simulink model "SimpleOrbitModel"  (R2025b)
settings: Solver=ode4  StartTime=0.0  StopTime=20000  FixedStep=60  RelTol=1e-3
undefined symbols (not defined in the file or in its folder): IAU, juliandate
libraries: aerolibtransform2 x1, aerolibatmos2 x1
settings Model: Creator=mbgm9nc4  LastModifiedBy=ewanb

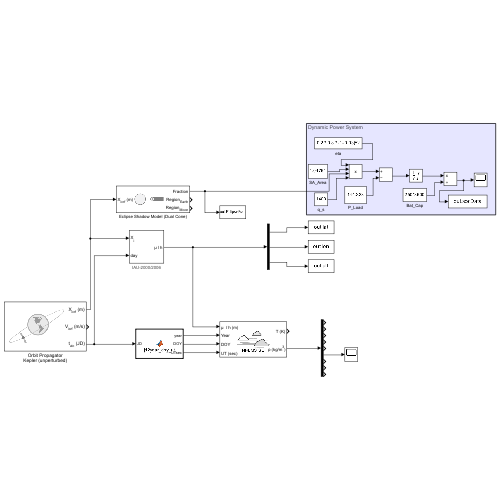
[thumbnail: Simulink's stored preview of the top-level diagram]
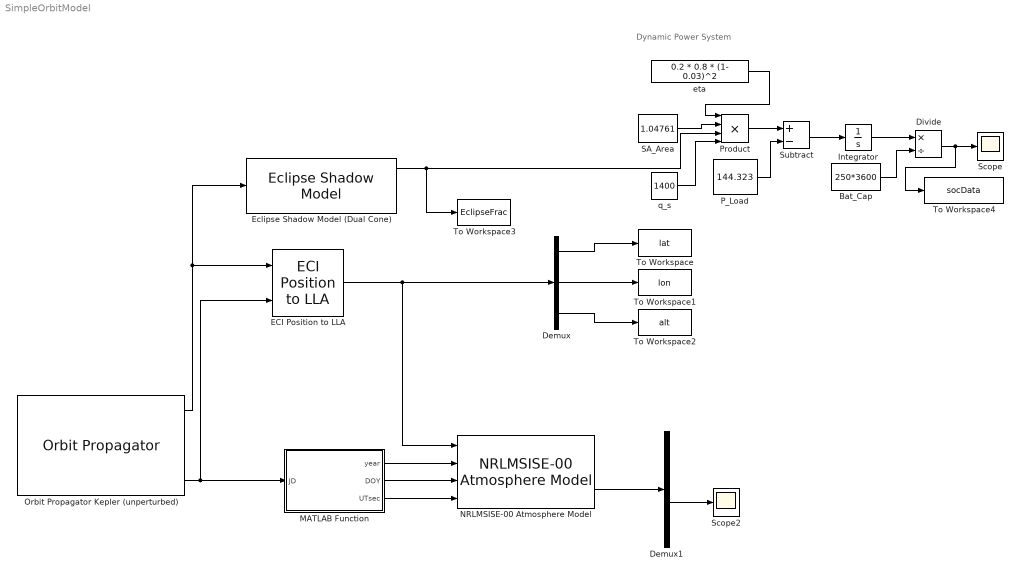
== system SimpleOrbitModel ==
  note: Dynamic Power System
  Bat_Cap : Constant  Value=250*3600
  Demux : Demux  Outputs=3
  Demux1 : Demux  Outputs=9
  Divide : Product  Inputs=*/
  ECI Position to LLA : aerolibtransform2/ECI Position to LLA  red=IAU-2000/2006  year=2013  month=January  day=1  hour=0  min=0  sec=0  deltaT=Day  errorflag=Error  extraparamflag=off  eunits=Metric (MKS)  earthmodel=WGS84  flat=1/298.257223563  eqradius=6378137
      settings: AttributesFormatString=%<red>
  Eclipse Shadow Model (Dual Cone) : EclipseShadowModel  shadowModel=Cylindrical  outputShadowRegion=on
  Integrator : Integrator  InitialCondition=250*3600  LimitOutput=on  UpperSaturationLimit=900000  LowerSaturationLimit=0
  MATLAB Function : MATLAB Function  TreatAsAtomicUnit=on
  NRLMSISE-00 Atmosphere Model : aerolibatmos2/NRLMSISE-00 Atmosphere Model  units=Metric (MKS)  lst_input=off  flux_ap_input=off  flags_input=Internal  flags=ones(1,23)  oxygen_in=off  action=Warning
  Orbit Propagator Kepler (unperturbed) : OrbitPropagator  startDate=juliandate(2026, 3, 20, 12, 0, 0)  semiMajorAxis=(6378+330.5)*1000  eccentricity=0  inclination=96.78  raan=337.5  argPeriapsis=0  trueAnomaly=0  inertialPosition=[3649700.0 3308200.0 -4676600.0]  inertialVelocity=[-2750.8 6666.4 2573.4]  fixedPosition=[-4142689.0 -2676864.7 -4669861.6]  fixedVelocity=[1452.7 -6720.7 2568.1]  customR=3396200  customMu=4.305e13  customJ2=1.0826269e-03  customOmega=4.06125949e-3
  P_Load : Constant  Value=144.323
  Product : Product  Inputs=4
  SA_Area : Constant  Value=1.04761
  Scope : Scope
      settings: ActiveDisplayYMinimum=0.72729250193319717  ActiveDisplayYMaximum=1.0075459538843075
  Scope2 : Scope
      settings: ActiveDisplayYMinimum=6.5102533120978795E-12  ActiveDisplayYMaximum=2.3152198434120581E-11
  Subtract : Sum  Inputs=+-
  To Workspace : ToWorkspace  VariableName=lat  SaveFormat=Timeseries  SampleTime=-1
  To Workspace1 : ToWorkspace  VariableName=lon  SaveFormat=Timeseries  SampleTime=-1
  To Workspace2 : ToWorkspace  VariableName=alt  SaveFormat=Timeseries  SampleTime=-1
  To Workspace3 : ToWorkspace  VariableName=EclipseFrac  SaveFormat=Timeseries  SampleTime=-1
  To Workspace4 : ToWorkspace  VariableName=socData  SampleTime=-1
  eta : Constant  Value=0.2 * 0.8 * (1- 0.03)^2
  q_s : Constant  Value=1400
  wires:
  Demux/2 -> To Workspace1/1
  q_s/1 -> Product/4
  Bat_Cap/1 -> Divide/2
  Subtract/1 -> Integrator/1
  Demux/3 -> To Workspace2/1
  eta/1 -> Product/1
  SA_Area/1 -> Product/2
  P_Load/1 -> Subtract/2
  Orbit Propagator Kepler (unperturbed)/1 -> Eclipse Shadow Model (Dual Cone)/1, ECI Position to LLA/1
  Product/1 -> Subtract/1
  MATLAB Function/2(DOY) -> NRLMSISE-00 Atmosphere Model/3
  Integrator/1 -> Divide/1
  ECI Position to LLA/1 -> NRLMSISE-00 Atmosphere Model/1, Demux/1
  Divide/1 -> To Workspace4/1, Scope/1
  Orbit Propagator Kepler (unperturbed)/3 -> ECI Position to LLA/2, MATLAB Function/1(JD)
  MATLAB Function/1(year) -> NRLMSISE-00 Atmosphere Model/2
  MATLAB Function/3(UTsec) -> NRLMSISE-00 Atmosphere Model/4
  Demux/1 -> To Workspace/1
  NRLMSISE-00 Atmosphere Model/2 -> Demux1/1
  Demux1/6 -> Scope2/1
  Eclipse Shadow Model (Dual Cone)/1 -> Product/3, To Workspace3/1

== matlab function SimpleOrbitModel/MATLAB Function ==
  data: year output; JD input; DOY output; UTsec output
function [year, DOY, UTsec] = jd2year_doy_ut(JD)
% Input:
%   JD   - Julian Date (UTC)
% Outputs:
%   year  - Gregorian year
%   DOY   - Day of year (1–366)
%   UTsec - Seconds past 00:00:00 UTC

% ---- Shift because JD starts at noon
JD_shift = JD + 0.5;
Z = floor(JD_shift);
F = JD_shift - Z;

% ---- UT seconds
UTsec = F * 86400.0;

% ---- Gregorian calendar conversion (Fliegel–Van Flandern)
alpha = floor((Z - 1867216.25)/36524.25);
A = Z + 1 + alpha - floor(alpha/4);
B = A + 1524;
C = floor((B - 122.1)/365.25);
D = floor(365.25 * C);
E = floor((B - D)/30.6001);
day = B - D - floor(30.6001 * E);

if E < 14
    month = E - 1;
else
    month = E - 13;
end

if month > 2
    year = C - 4716;
else
    year = C - 4715;
end

% ---- Compute DOY
% Leap year test
isLeap = (mod(year,4)==0 && mod(year,100)~=0) || mod(year,400)==0;
monthDays = [31 28+isLeap 31 30 31 30 31 31 30 31 30 31];
DOY = day;
for k = 1:month-1
    DOY = DOY + monthDays(k);
end

end
